simulink model "21-E"  (R2014a)
settings: Solver=FixedStepDiscrete  StartTime=0.0  StopTime=10.0  FixedStep=0.0005  RelTol=1e-3
undefined symbols (not defined in the file): add_k1_100, add_k2_100, ADDspeed, cal_acc_div, cal_acc_flo_add, cal_acc_min, cal_an_div, cal_an_min, cal_bre_div, cal_bre_en_add, cal_bre_flo_add, cal_bre_min, cal_conf_off, cal_conf_on, controller, ecucoder_acal, enres_on_add, enres_per_add
libraries: simulink x165, ec55xxlib x29
(part 2 of 6)

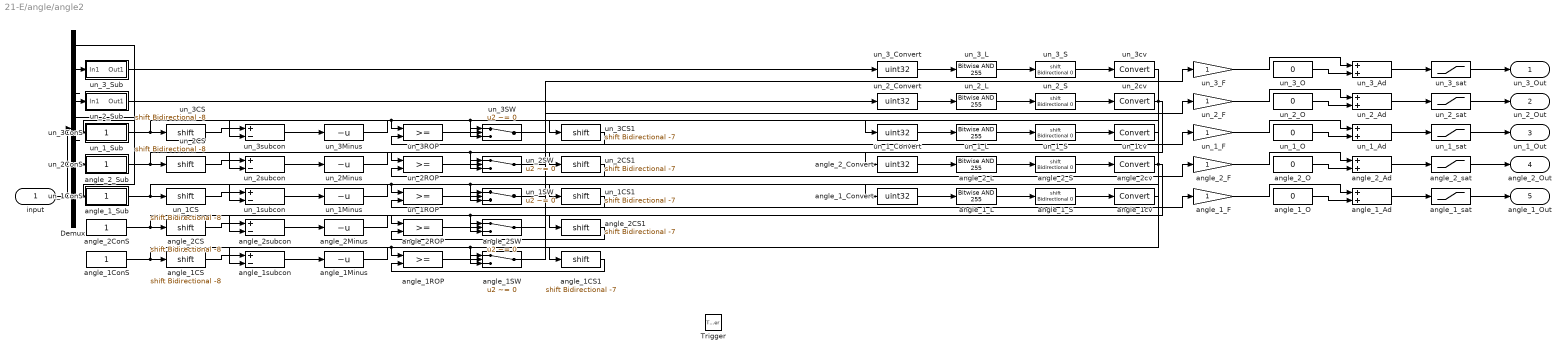
== system 21-E/angle/angle2 ==
  input : Inport
  Trigger : TriggerPort  TriggerType=function-call  PortDimensions=1
  Demux : Demux  Outputs=8
  angle_1CS : ArithShift  BitShiftNumber=-8
  angle_1CS1 : ArithShift  BitShiftNumber=-7
  angle_1ConS : Constant  OutDataTypeStr=single
  angle_1Minus : UnaryMinus
  angle_1ROP : RelationalOperator  OutDataTypeStr=boolean
  angle_1SW : Switch  Criteria=u2 ~= 0
  angle_1_Ad : Sum
  angle_1_Convert : DataTypeConversion  OutDataTypeStr=uint32
  angle_1_F : Gain
  angle_1_L : simulink/Logic and Bit Operations/Bitwise Operator  logicop=AND  UseBitMask=on  BitMask=255  BitMaskRealWorld=Stored Integer
  angle_1_O : Constant  Value=0  OutDataTypeStr=single
  angle_1_S : ArithShift
  angle_1_Sub : Subsystem
  angle_1_sat : Saturate  UpperLimit=255  LowerLimit=0
  angle_1cv : DataTypeConversion
  angle_1subcon : Sum  Inputs=+-
  angle_2CS : ArithShift  BitShiftNumber=-8
  angle_2CS1 : ArithShift  BitShiftNumber=-7
  angle_2ConS : Constant  OutDataTypeStr=single
  angle_2Minus : UnaryMinus
  angle_2ROP : RelationalOperator  OutDataTypeStr=boolean
  angle_2SW : Switch  Criteria=u2 ~= 0
  angle_2_Ad : Sum
  angle_2_Convert : DataTypeConversion  OutDataTypeStr=uint32
  angle_2_F : Gain
  angle_2_L : simulink/Logic and Bit Operations/Bitwise Operator  logicop=AND  UseBitMask=on  BitMask=255  BitMaskRealWorld=Stored Integer
  angle_2_O : Constant  Value=0  OutDataTypeStr=single
  angle_2_S : ArithShift
  angle_2_Sub : Subsystem
  angle_2_sat : Saturate  UpperLimit=255  LowerLimit=0
  angle_2cv : DataTypeConversion
  angle_2subcon : Sum  Inputs=+-
  un_1CS : ArithShift  BitShiftNumber=-8
  un_1CS1 : ArithShift  BitShiftNumber=-7
  un_1ConS : Constant  OutDataTypeStr=single
  un_1Minus : UnaryMinus
  un_1ROP : RelationalOperator  OutDataTypeStr=boolean
  un_1SW : Switch  Criteria=u2 ~= 0
  un_1_Ad : Sum
  un_1_Convert : DataTypeConversion  OutDataTypeStr=uint32
  un_1_F : Gain
  un_1_L : simulink/Logic and Bit Operations/Bitwise Operator  logicop=AND  UseBitMask=on  BitMask=255  BitMaskRealWorld=Stored Integer
  un_1_O : Constant  Value=0  OutDataTypeStr=single
  un_1_S : ArithShift
  un_1_Sub : Subsystem
  un_1_sat : Saturate  UpperLimit=255  LowerLimit=0
  un_1cv : DataTypeConversion
  un_1subcon : Sum  Inputs=+-
  un_2CS : ArithShift  BitShiftNumber=-8
  un_2CS1 : ArithShift  BitShiftNumber=-7
  un_2ConS : Constant  OutDataTypeStr=single
  un_2Minus : UnaryMinus
  un_2ROP : RelationalOperator  OutDataTypeStr=boolean
  un_2SW : Switch  Criteria=u2 ~= 0
  un_2_Ad : Sum
  un_2_Convert : DataTypeConversion  OutDataTypeStr=uint32
  un_2_F : Gain
  un_2_L : simulink/Logic and Bit Operations/Bitwise Operator  logicop=AND  UseBitMask=on  BitMask=255  BitMaskRealWorld=Stored Integer
  un_2_O : Constant  Value=0  OutDataTypeStr=single
  un_2_S : ArithShift
  un_2_Sub : Subsystem
  un_2_sat : Saturate  UpperLimit=255  LowerLimit=0
  un_2cv : DataTypeConversion
  un_2subcon : Sum  Inputs=+-
  un_3CS : ArithShift  BitShiftNumber=-8
  un_3CS1 : ArithShift  BitShiftNumber=-7
  un_3ConS : Constant  OutDataTypeStr=single
  un_3Minus : UnaryMinus
  un_3ROP : RelationalOperator  OutDataTypeStr=boolean
  un_3SW : Switch  Criteria=u2 ~= 0
  un_3_Ad : Sum
  un_3_Convert : DataTypeConversion  OutDataTypeStr=uint32
  un_3_F : Gain
  un_3_L : simulink/Logic and Bit Operations/Bitwise Operator  logicop=AND  UseBitMask=on  BitMask=255  BitMaskRealWorld=Stored Integer
  un_3_O : Constant  Value=0  OutDataTypeStr=single
  un_3_S : ArithShift
  un_3_Sub : Subsystem
  un_3_sat : Saturate  UpperLimit=255  LowerLimit=0
  un_3cv : DataTypeConversion
  un_3subcon : Sum  Inputs=+-
  un_3_Out : Outport
  un_2_Out : Outport  Port=2
  un_1_Out : Outport  Port=3
  angle_2_Out : Outport  Port=4
  angle_1_Out : Outport  Port=5
  wires:
  input/1 -> Demux/1
  angle_1ROP/1 -> angle_1SW/2
  angle_1SW/1 -> angle_1_F/1
  angle_1Minus/1 -> angle_1SW/1
  angle_1subcon/1 -> angle_1Minus/1
  angle_1CS/1 -> angle_1subcon/1
  angle_1CS1/1 -> angle_1ROP/2
  angle_1ConS/1 -> angle_1CS1/1, angle_1CS/1
  angle_1cv/1 -> angle_1subcon/2, angle_1ROP/1, angle_1SW/3
  angle_1_S/1 -> angle_1cv/1
  angle_1_L/1 -> angle_1_S/1
  angle_1_Convert/1 -> angle_1_L/1
  angle_1_Sub/1(Out1) -> angle_1_Convert/1
  Demux/4 -> angle_1_Sub/1(In1)
  angle_1_sat/1 -> angle_1_Out/1
  angle_1_Ad/1 -> angle_1_sat/1
  angle_1_O/1 -> angle_1_Ad/2
  angle_1_F/1 -> angle_1_Ad/1
  angle_2ROP/1 -> angle_2SW/2
  angle_2SW/1 -> angle_2_F/1
  angle_2Minus/1 -> angle_2SW/1
  angle_2subcon/1 -> angle_2Minus/1
  angle_2CS/1 -> angle_2subcon/1
  angle_2CS1/1 -> angle_2ROP/2
  angle_2ConS/1 -> angle_2CS1/1, angle_2CS/1
  angle_2cv/1 -> angle_2SW/3, angle_2subcon/2, angle_2ROP/1
  angle_2_S/1 -> angle_2cv/1
  angle_2_L/1 -> angle_2_S/1
  angle_2_Convert/1 -> angle_2_L/1
  angle_2_Sub/1(Out1) -> angle_2_Convert/1
  Demux/5 -> angle_2_Sub/1(In1)
  angle_2_sat/1 -> angle_2_Out/1
  angle_2_Ad/1 -> angle_2_sat/1
  angle_2_O/1 -> angle_2_Ad/2
  angle_2_F/1 -> angle_2_Ad/1
  un_1ROP/1 -> un_1SW/2
  un_1SW/1 -> un_1_F/1
  un_1Minus/1 -> un_1SW/1
  un_1subcon/1 -> un_1Minus/1
  un_1CS/1 -> un_1subcon/1
  un_1CS1/1 -> un_1ROP/2
  un_1ConS/1 -> un_1CS1/1, un_1CS/1
  un_1cv/1 -> un_1subcon/2, un_1ROP/1, un_1SW/3
  un_1_S/1 -> un_1cv/1
  un_1_L/1 -> un_1_S/1
  un_1_Convert/1 -> un_1_L/1
  un_1_Sub/1(Out1) -> un_1_Convert/1
  Demux/1 -> un_1_Sub/1(In1)
  un_1_sat/1 -> un_1_Out/1
  un_1_Ad/1 -> un_1_sat/1
  un_1_O/1 -> un_1_Ad/2
  un_1_F/1 -> un_1_Ad/1
  un_2ROP/1 -> un_2SW/2
  un_2SW/1 -> un_2_F/1
  un_2Minus/1 -> un_2SW/1
  un_2subcon/1 -> un_2Minus/1
  un_2CS/1 -> un_2subcon/1
  un_2CS1/1 -> un_2ROP/2
  un_2ConS/1 -> un_2CS1/1, un_2CS/1
  un_2cv/1 -> un_2SW/3, un_2subcon/2, un_2ROP/1
  un_2_S/1 -> un_2cv/1
  un_2_L/1 -> un_2_S/1
  un_2_Convert/1 -> un_2_L/1
  un_2_Sub/1(Out1) -> un_2_Convert/1
  Demux/2 -> un_2_Sub/1(In1)
  un_2_sat/1 -> un_2_Out/1
  un_2_Ad/1 -> un_2_sat/1
  un_2_O/1 -> un_2_Ad/2
  un_2_F/1 -> un_2_Ad/1
  un_3ROP/1 -> un_3SW/2
  un_3SW/1 -> un_3_F/1
  un_3Minus/1 -> un_3SW/1
  un_3subcon/1 -> un_3Minus/1
  un_3CS/1 -> un_3subcon/1
  un_3CS1/1 -> un_3ROP/2
  un_3ConS/1 -> un_3CS1/1, un_3CS/1
  un_3cv/1 -> un_3subcon/2, un_3ROP/1, un_3SW/3
  un_3_S/1 -> un_3cv/1
  un_3_L/1 -> un_3_S/1
  un_3_Convert/1 -> un_3_L/1
  un_3_Sub/1(Out1) -> un_3_Convert/1
  Demux/3 -> un_3_Sub/1(In1)
  un_3_sat/1 -> un_3_Out/1
  un_3_Ad/1 -> un_3_sat/1
  un_3_O/1 -> un_3_Ad/2
  un_3_F/1 -> un_3_Ad/1

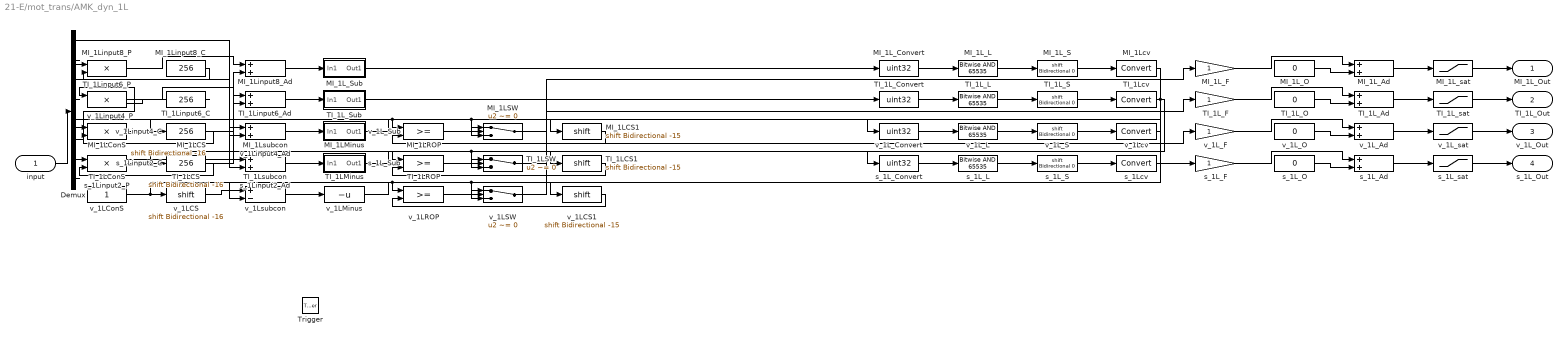
== system 21-E/mot_trans/AMK_dyn_1L ==
  input : Inport
  Trigger : TriggerPort  TriggerType=function-call  PortDimensions=1
  Demux : Demux  Outputs=8
  MI_1LCS : ArithShift  BitShiftNumber=-16
  MI_1LCS1 : ArithShift  BitShiftNumber=-15
  MI_1LConS : Constant  OutDataTypeStr=single
  MI_1LMinus : UnaryMinus
  MI_1LROP : RelationalOperator  OutDataTypeStr=boolean
  MI_1LSW : Switch  Criteria=u2 ~= 0
  MI_1L_Ad : Sum
  MI_1L_Convert : DataTypeConversion  OutDataTypeStr=uint32
  MI_1L_F : Gain
  MI_1L_L : simulink/Logic and Bit Operations/Bitwise Operator  logicop=AND  UseBitMask=on  BitMask=65535  BitMaskRealWorld=Stored Integer
  MI_1L_O : Constant  Value=0  OutDataTypeStr=single
  MI_1L_S : ArithShift
  MI_1L_Sub : Subsystem
  MI_1L_sat : Saturate  UpperLimit=32767  LowerLimit=-32768
  MI_1Lcv : DataTypeConversion
  MI_1Linput8_Ad : Sum
  MI_1Linput8_C : Constant  Value=256
  MI_1Linput8_P : Product
  MI_1Lsubcon : Sum  Inputs=+-
  TI_1LCS : ArithShift  BitShiftNumber=-16
  TI_1LCS1 : ArithShift  BitShiftNumber=-15
  TI_1LConS : Constant  OutDataTypeStr=single
  TI_1LMinus : UnaryMinus
  TI_1LROP : RelationalOperator  OutDataTypeStr=boolean
  TI_1LSW : Switch  Criteria=u2 ~= 0
  TI_1L_Ad : Sum
  TI_1L_Convert : DataTypeConversion  OutDataTypeStr=uint32
  TI_1L_F : Gain
  TI_1L_L : simulink/Logic and Bit Operations/Bitwise Operator  logicop=AND  UseBitMask=on  BitMask=65535  BitMaskRealWorld=Stored Integer
  TI_1L_O : Constant  Value=0  OutDataTypeStr=single
  TI_1L_S : ArithShift
  TI_1L_Sub : Subsystem
  TI_1L_sat : Saturate  UpperLimit=32767  LowerLimit=-32768
  TI_1Lcv : DataTypeConversion
  TI_1Linput6_Ad : Sum
  TI_1Linput6_C : Constant  Value=256
  TI_1Linput6_P : Product
  TI_1Lsubcon : Sum  Inputs=+-
  s_1L_Ad : Sum
  s_1L_Convert : DataTypeConversion  OutDataTypeStr=uint32
  s_1L_F : Gain
  s_1L_L : simulink/Logic and Bit Operations/Bitwise Operator  logicop=AND  UseBitMask=on  BitMask=65535  BitMaskRealWorld=Stored Integer
  s_1L_O : Constant  Value=0  OutDataTypeStr=single
  s_1L_S : ArithShift
  s_1L_Sub : Subsystem
  s_1L_sat : Saturate  UpperLimit=65535  LowerLimit=0
  s_1Lcv : DataTypeConversion
  s_1Linput2_Ad : Sum
  s_1Linput2_C : Constant  Value=256
  s_1Linput2_P : Product
  v_1LCS : ArithShift  BitShiftNumber=-16
  v_1LCS1 : ArithShift  BitShiftNumber=-15
  v_1LConS : Constant  OutDataTypeStr=single
  v_1LMinus : UnaryMinus
  v_1LROP : RelationalOperator  OutDataTypeStr=boolean
  v_1LSW : Switch  Criteria=u2 ~= 0
  v_1L_Ad : Sum
  v_1L_Convert : DataTypeConversion  OutDataTypeStr=uint32
  v_1L_F : Gain
  v_1L_L : simulink/Logic and Bit Operations/Bitwise Operator  logicop=AND  UseBitMask=on  BitMask=65535  BitMaskRealWorld=Stored Integer
  v_1L_O : Constant  Value=0  OutDataTypeStr=single
  v_1L_S : ArithShift
  v_1L_Sub : Subsystem
  v_1L_sat : Saturate  UpperLimit=32767  LowerLimit=-32768
  v_1Lcv : DataTypeConversion
  v_1Linput4_Ad : Sum
  v_1Linput4_C : Constant  Value=256
  v_1Linput4_P : Product
  v_1Lsubcon : Sum  Inputs=+-
  MI_1L_Out : Outport
  TI_1L_Out : Outport  Port=2
  v_1L_Out : Outport  Port=3
  s_1L_Out : Outport  Port=4
  wires:
  input/1 -> Demux/1
  s_1Lcv/1 -> s_1L_F/1
  s_1L_S/1 -> s_1Lcv/1
  s_1L_L/1 -> s_1L_S/1
  s_1L_Convert/1 -> s_1L_L/1
  s_1L_Sub/1(Out1) -> s_1L_Convert/1
  s_1Linput2_Ad/1 -> s_1L_Sub/1(In1)
  Demux/1 -> s_1Linput2_Ad/2
  s_1Linput2_P/1 -> s_1Linput2_Ad/1
  s_1Linput2_C/1 -> s_1Linput2_P/2
  Demux/2 -> s_1Linput2_P/1
  s_1L_sat/1 -> s_1L_Out/1
  s_1L_Ad/1 -> s_1L_sat/1
  s_1L_O/1 -> s_1L_Ad/2
  s_1L_F/1 -> s_1L_Ad/1
  v_1LROP/1 -> v_1LSW/2
  v_1LSW/1 -> v_1L_F/1
  v_1LMinus/1 -> v_1LSW/1
  v_1Lsubcon/1 -> v_1LMinus/1
  v_1LCS/1 -> v_1Lsubcon/1
  v_1LCS1/1 -> v_1LROP/2
  v_1LConS/1 -> v_1LCS1/1, v_1LCS/1
  v_1Lcv/1 -> v_1Lsubcon/2, v_1LROP/1, v_1LSW/3
  v_1L_S/1 -> v_1Lcv/1
  v_1L_L/1 -> v_1L_S/1
  v_1L_Convert/1 -> v_1L_L/1
  v_1L_Sub/1(Out1) -> v_1L_Convert/1
  v_1Linput4_Ad/1 -> v_1L_Sub/1(In1)
  Demux/3 -> v_1Linput4_Ad/2
  v_1Linput4_P/1 -> v_1Linput4_Ad/1
  v_1Linput4_C/1 -> v_1Linput4_P/2
  Demux/4 -> v_1Linput4_P/1
  v_1L_sat/1 -> v_1L_Out/1
  v_1L_Ad/1 -> v_1L_sat/1
  v_1L_O/1 -> v_1L_Ad/2
  v_1L_F/1 -> v_1L_Ad/1
  TI_1LROP/1 -> TI_1LSW/2
  TI_1LSW/1 -> TI_1L_F/1
  TI_1LMinus/1 -> TI_1LSW/1
  TI_1Lsubcon/1 -> TI_1LMinus/1
  TI_1LCS/1 -> TI_1Lsubcon/1
  TI_1LCS1/1 -> TI_1LROP/2
  TI_1LConS/1 -> TI_1LCS1/1, TI_1LCS/1
  TI_1Lcv/1 -> TI_1LSW/3, TI_1Lsubcon/2, TI_1LROP/1
  TI_1L_S/1 -> TI_1Lcv/1
  TI_1L_L/1 -> TI_1L_S/1
  TI_1L_Convert/1 -> TI_1L_L/1
  TI_1L_Sub/1(Out1) -> TI_1L_Convert/1
  TI_1Linput6_Ad/1 -> TI_1L_Sub/1(In1)
  Demux/5 -> TI_1Linput6_Ad/2
  TI_1Linput6_P/1 -> TI_1Linput6_Ad/1
  TI_1Linput6_C/1 -> TI_1Linput6_P/2
  Demux/6 -> TI_1Linput6_P/1
  TI_1L_sat/1 -> TI_1L_Out/1
  TI_1L_Ad/1 -> TI_1L_sat/1
  TI_1L_O/1 -> TI_1L_Ad/2
  TI_1L_F/1 -> TI_1L_Ad/1
  MI_1LROP/1 -> MI_1LSW/2
  MI_1LSW/1 -> MI_1L_F/1
  MI_1LMinus/1 -> MI_1LSW/1
  MI_1Lsubcon/1 -> MI_1LMinus/1
  MI_1LCS/1 -> MI_1Lsubcon/1
  MI_1LCS1/1 -> MI_1LROP/2
  MI_1LConS/1 -> MI_1LCS1/1, MI_1LCS/1
  MI_1Lcv/1 -> MI_1Lsubcon/2, MI_1LROP/1, MI_1LSW/3
  MI_1L_S/1 -> MI_1Lcv/1
  MI_1L_L/1 -> MI_1L_S/1
  MI_1L_Convert/1 -> MI_1L_L/1
  MI_1L_Sub/1(Out1) -> MI_1L_Convert/1
  MI_1Linput8_Ad/1 -> MI_1L_Sub/1(In1)
  Demux/7 -> MI_1Linput8_Ad/2
  MI_1Linput8_P/1 -> MI_1Linput8_Ad/1
  MI_1Linput8_C/1 -> MI_1Linput8_P/2
  Demux/8 -> MI_1Linput8_P/1
  MI_1L_sat/1 -> MI_1L_Out/1
  MI_1L_Ad/1 -> MI_1L_sat/1
  MI_1L_O/1 -> MI_1L_Ad/2
  MI_1L_F/1 -> MI_1L_Ad/1

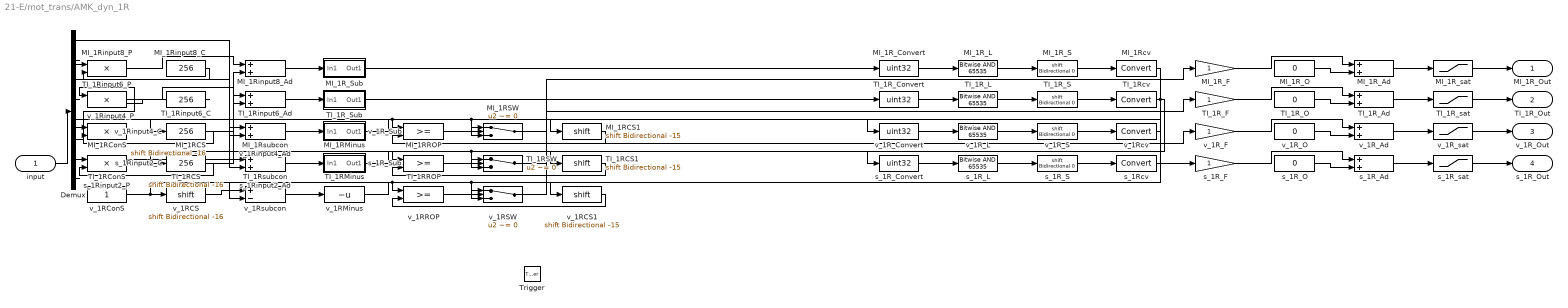
== system 21-E/mot_trans/AMK_dyn_1R ==
  input : Inport
  Trigger : TriggerPort  TriggerType=function-call  PortDimensions=1
  Demux : Demux  Outputs=8
  MI_1RCS : ArithShift  BitShiftNumber=-16
  MI_1RCS1 : ArithShift  BitShiftNumber=-15
  MI_1RConS : Constant  OutDataTypeStr=single
  MI_1RMinus : UnaryMinus
  MI_1RROP : RelationalOperator  OutDataTypeStr=boolean
  MI_1RSW : Switch  Criteria=u2 ~= 0
  MI_1R_Ad : Sum
  MI_1R_Convert : DataTypeConversion  OutDataTypeStr=uint32
  MI_1R_F : Gain
  MI_1R_L : simulink/Logic and Bit Operations/Bitwise Operator  logicop=AND  UseBitMask=on  BitMask=65535  BitMaskRealWorld=Stored Integer
  MI_1R_O : Constant  Value=0  OutDataTypeStr=single
  MI_1R_S : ArithShift
  MI_1R_Sub : Subsystem
  MI_1R_sat : Saturate  UpperLimit=32767  LowerLimit=-32768
  MI_1Rcv : DataTypeConversion
  MI_1Rinput8_Ad : Sum
  MI_1Rinput8_C : Constant  Value=256
  MI_1Rinput8_P : Product
  MI_1Rsubcon : Sum  Inputs=+-
  TI_1RCS : ArithShift  BitShiftNumber=-16
  TI_1RCS1 : ArithShift  BitShiftNumber=-15
  TI_1RConS : Constant  OutDataTypeStr=single
  TI_1RMinus : UnaryMinus
  TI_1RROP : RelationalOperator  OutDataTypeStr=boolean
  TI_1RSW : Switch  Criteria=u2 ~= 0
  TI_1R_Ad : Sum
  TI_1R_Convert : DataTypeConversion  OutDataTypeStr=uint32
  TI_1R_F : Gain
  TI_1R_L : simulink/Logic and Bit Operations/Bitwise Operator  logicop=AND  UseBitMask=on  BitMask=65535  BitMaskRealWorld=Stored Integer
  TI_1R_O : Constant  Value=0  OutDataTypeStr=single
  TI_1R_S : ArithShift
  TI_1R_Sub : Subsystem
  TI_1R_sat : Saturate  UpperLimit=32767  LowerLimit=-32768
  TI_1Rcv : DataTypeConversion
  TI_1Rinput6_Ad : Sum
  TI_1Rinput6_C : Constant  Value=256
  TI_1Rinput6_P : Product
  TI_1Rsubcon : Sum  Inputs=+-
  s_1R_Ad : Sum
  s_1R_Convert : DataTypeConversion  OutDataTypeStr=uint32
  s_1R_F : Gain
  s_1R_L : simulink/Logic and Bit Operations/Bitwise Operator  logicop=AND  UseBitMask=on  BitMask=65535  BitMaskRealWorld=Stored Integer
  s_1R_O : Constant  Value=0  OutDataTypeStr=single
  s_1R_S : ArithShift
  s_1R_Sub : Subsystem
  s_1R_sat : Saturate  UpperLimit=65535  LowerLimit=0
  s_1Rcv : DataTypeConversion
  s_1Rinput2_Ad : Sum
  s_1Rinput2_C : Constant  Value=256
  s_1Rinput2_P : Product
  v_1RCS : ArithShift  BitShiftNumber=-16
  v_1RCS1 : ArithShift  BitShiftNumber=-15
  v_1RConS : Constant  OutDataTypeStr=single
  v_1RMinus : UnaryMinus
  v_1RROP : RelationalOperator  OutDataTypeStr=boolean
  v_1RSW : Switch  Criteria=u2 ~= 0
  v_1R_Ad : Sum
  v_1R_Convert : DataTypeConversion  OutDataTypeStr=uint32
  v_1R_F : Gain
  v_1R_L : simulink/Logic and Bit Operations/Bitwise Operator  logicop=AND  UseBitMask=on  BitMask=65535  BitMaskRealWorld=Stored Integer
  v_1R_O : Constant  Value=0  OutDataTypeStr=single
  v_1R_S : ArithShift
  v_1R_Sub : Subsystem
  v_1R_sat : Saturate  UpperLimit=32767  LowerLimit=-32768
  v_1Rcv : DataTypeConversion
  v_1Rinput4_Ad : Sum
  v_1Rinput4_C : Constant  Value=256
  v_1Rinput4_P : Product
  v_1Rsubcon : Sum  Inputs=+-
  MI_1R_Out : Outport
  TI_1R_Out : Outport  Port=2
  v_1R_Out : Outport  Port=3
  s_1R_Out : Outport  Port=4
  wires:
  input/1 -> Demux/1
  s_1Rcv/1 -> s_1R_F/1
  s_1R_S/1 -> s_1Rcv/1
  s_1R_L/1 -> s_1R_S/1
  s_1R_Convert/1 -> s_1R_L/1
  s_1R_Sub/1(Out1) -> s_1R_Convert/1
  s_1Rinput2_Ad/1 -> s_1R_Sub/1(In1)
  Demux/1 -> s_1Rinput2_Ad/2
  s_1Rinput2_P/1 -> s_1Rinput2_Ad/1
  s_1Rinput2_C/1 -> s_1Rinput2_P/2
  Demux/2 -> s_1Rinput2_P/1
  s_1R_sat/1 -> s_1R_Out/1
  s_1R_Ad/1 -> s_1R_sat/1
  s_1R_O/1 -> s_1R_Ad/2
  s_1R_F/1 -> s_1R_Ad/1
  v_1RROP/1 -> v_1RSW/2
  v_1RSW/1 -> v_1R_F/1
  v_1RMinus/1 -> v_1RSW/1
  v_1Rsubcon/1 -> v_1RMinus/1
  v_1RCS/1 -> v_1Rsubcon/1
  v_1RCS1/1 -> v_1RROP/2
  v_1RConS/1 -> v_1RCS1/1, v_1RCS/1
  v_1Rcv/1 -> v_1Rsubcon/2, v_1RROP/1, v_1RSW/3
  v_1R_S/1 -> v_1Rcv/1
  v_1R_L/1 -> v_1R_S/1
  v_1R_Convert/1 -> v_1R_L/1
  v_1R_Sub/1(Out1) -> v_1R_Convert/1
  v_1Rinput4_Ad/1 -> v_1R_Sub/1(In1)
  Demux/3 -> v_1Rinput4_Ad/2
  v_1Rinput4_P/1 -> v_1Rinput4_Ad/1
  v_1Rinput4_C/1 -> v_1Rinput4_P/2
  Demux/4 -> v_1Rinput4_P/1
  v_1R_sat/1 -> v_1R_Out/1
  v_1R_Ad/1 -> v_1R_sat/1
  v_1R_O/1 -> v_1R_Ad/2
  v_1R_F/1 -> v_1R_Ad/1
  TI_1RROP/1 -> TI_1RSW/2
  TI_1RSW/1 -> TI_1R_F/1
  TI_1RMinus/1 -> TI_1RSW/1
  TI_1Rsubcon/1 -> TI_1RMinus/1
  TI_1RCS/1 -> TI_1Rsubcon/1
  TI_1RCS1/1 -> TI_1RROP/2
  TI_1RConS/1 -> TI_1RCS1/1, TI_1RCS/1
  TI_1Rcv/1 -> TI_1RSW/3, TI_1Rsubcon/2, TI_1RROP/1
  TI_1R_S/1 -> TI_1Rcv/1
  TI_1R_L/1 -> TI_1R_S/1
  TI_1R_Convert/1 -> TI_1R_L/1
  TI_1R_Sub/1(Out1) -> TI_1R_Convert/1
  TI_1Rinput6_Ad/1 -> TI_1R_Sub/1(In1)
  Demux/5 -> TI_1Rinput6_Ad/2
  TI_1Rinput6_P/1 -> TI_1Rinput6_Ad/1
  TI_1Rinput6_C/1 -> TI_1Rinput6_P/2
  Demux/6 -> TI_1Rinput6_P/1
  TI_1R_sat/1 -> TI_1R_Out/1
  TI_1R_Ad/1 -> TI_1R_sat/1
  TI_1R_O/1 -> TI_1R_Ad/2
  TI_1R_F/1 -> TI_1R_Ad/1
  MI_1RROP/1 -> MI_1RSW/2
  MI_1RSW/1 -> MI_1R_F/1
  MI_1RMinus/1 -> MI_1RSW/1
  MI_1Rsubcon/1 -> MI_1RMinus/1
  MI_1RCS/1 -> MI_1Rsubcon/1
  MI_1RCS1/1 -> MI_1RROP/2
  MI_1RConS/1 -> MI_1RCS1/1, MI_1RCS/1
  MI_1Rcv/1 -> MI_1Rsubcon/2, MI_1RROP/1, MI_1RSW/3
  MI_1R_S/1 -> MI_1Rcv/1
  MI_1R_L/1 -> MI_1R_S/1
  MI_1R_Convert/1 -> MI_1R_L/1
  MI_1R_Sub/1(Out1) -> MI_1R_Convert/1
  MI_1Rinput8_Ad/1 -> MI_1R_Sub/1(In1)
  Demux/7 -> MI_1Rinput8_Ad/2
  MI_1Rinput8_P/1 -> MI_1Rinput8_Ad/1
  MI_1Rinput8_C/1 -> MI_1Rinput8_P/2
  Demux/8 -> MI_1Rinput8_P/1
  MI_1R_sat/1 -> MI_1R_Out/1
  MI_1R_Ad/1 -> MI_1R_sat/1
  MI_1R_O/1 -> MI_1R_Ad/2
  MI_1R_F/1 -> MI_1R_Ad/1

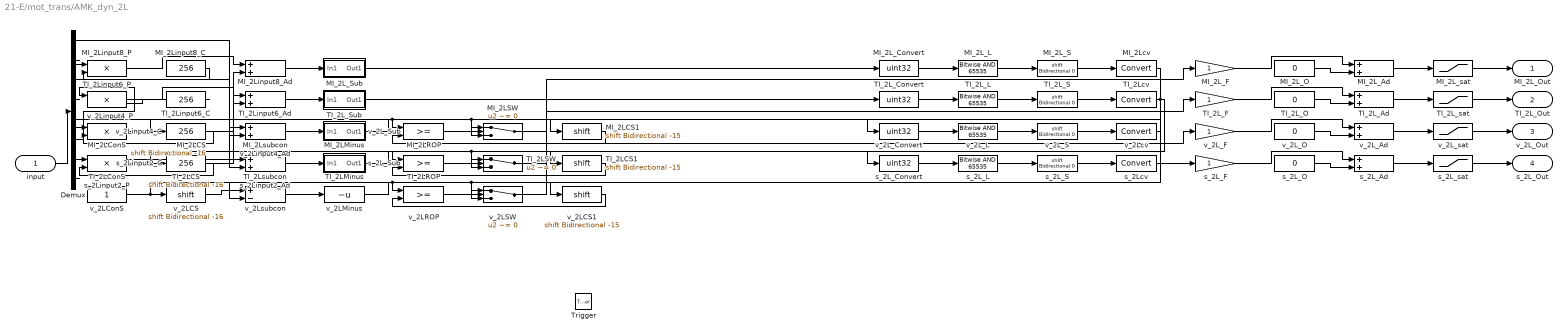
== system 21-E/mot_trans/AMK_dyn_2L ==
  input : Inport
  Trigger : TriggerPort  TriggerType=function-call  PortDimensions=1
  Demux : Demux  Outputs=8
  MI_2LCS : ArithShift  BitShiftNumber=-16
  MI_2LCS1 : ArithShift  BitShiftNumber=-15
  MI_2LConS : Constant  OutDataTypeStr=single
  MI_2LMinus : UnaryMinus
  MI_2LROP : RelationalOperator  OutDataTypeStr=boolean
  MI_2LSW : Switch  Criteria=u2 ~= 0
  MI_2L_Ad : Sum
  MI_2L_Convert : DataTypeConversion  OutDataTypeStr=uint32
  MI_2L_F : Gain
  MI_2L_L : simulink/Logic and Bit Operations/Bitwise Operator  logicop=AND  UseBitMask=on  BitMask=65535  BitMaskRealWorld=Stored Integer
  MI_2L_O : Constant  Value=0  OutDataTypeStr=single
  MI_2L_S : ArithShift
  MI_2L_Sub : Subsystem
  MI_2L_sat : Saturate  UpperLimit=32767  LowerLimit=-32768
  MI_2Lcv : DataTypeConversion
  MI_2Linput8_Ad : Sum
  MI_2Linput8_C : Constant  Value=256
  MI_2Linput8_P : Product
  MI_2Lsubcon : Sum  Inputs=+-
  TI_2LCS : ArithShift  BitShiftNumber=-16
  TI_2LCS1 : ArithShift  BitShiftNumber=-15
  TI_2LConS : Constant  OutDataTypeStr=single
  TI_2LMinus : UnaryMinus
  TI_2LROP : RelationalOperator  OutDataTypeStr=boolean
  TI_2LSW : Switch  Criteria=u2 ~= 0
  TI_2L_Ad : Sum
  TI_2L_Convert : DataTypeConversion  OutDataTypeStr=uint32
  TI_2L_F : Gain
  TI_2L_L : simulink/Logic and Bit Operations/Bitwise Operator  logicop=AND  UseBitMask=on  BitMask=65535  BitMaskRealWorld=Stored Integer
  TI_2L_O : Constant  Value=0  OutDataTypeStr=single
  TI_2L_S : ArithShift
  TI_2L_Sub : Subsystem
  TI_2L_sat : Saturate  UpperLimit=32767  LowerLimit=-32768
  TI_2Lcv : DataTypeConversion
  TI_2Linput6_Ad : Sum
  TI_2Linput6_C : Constant  Value=256
  TI_2Linput6_P : Product
  TI_2Lsubcon : Sum  Inputs=+-
  s_2L_Ad : Sum
  s_2L_Convert : DataTypeConversion  OutDataTypeStr=uint32
  s_2L_F : Gain
  s_2L_L : simulink/Logic and Bit Operations/Bitwise Operator  logicop=AND  UseBitMask=on  BitMask=65535  BitMaskRealWorld=Stored Integer
  s_2L_O : Constant  Value=0  OutDataTypeStr=single
  s_2L_S : ArithShift
  s_2L_Sub : Subsystem
  s_2L_sat : Saturate  UpperLimit=65535  LowerLimit=0
  s_2Lcv : DataTypeConversion
  s_2Linput2_Ad : Sum
  s_2Linput2_C : Constant  Value=256
  s_2Linput2_P : Product
  v_2LCS : ArithShift  BitShiftNumber=-16
  v_2LCS1 : ArithShift  BitShiftNumber=-15
  v_2LConS : Constant  OutDataTypeStr=single
  v_2LMinus : UnaryMinus
  v_2LROP : RelationalOperator  OutDataTypeStr=boolean
  v_2LSW : Switch  Criteria=u2 ~= 0
  v_2L_Ad : Sum
  v_2L_Convert : DataTypeConversion  OutDataTypeStr=uint32
  v_2L_F : Gain
  v_2L_L : simulink/Logic and Bit Operations/Bitwise Operator  logicop=AND  UseBitMask=on  BitMask=65535  BitMaskRealWorld=Stored Integer
  v_2L_O : Constant  Value=0  OutDataTypeStr=single
  v_2L_S : ArithShift
  v_2L_Sub : Subsystem
  v_2L_sat : Saturate  UpperLimit=32767  LowerLimit=-32768
  v_2Lcv : DataTypeConversion
  v_2Linput4_Ad : Sum
  v_2Linput4_C : Constant  Value=256
  v_2Linput4_P : Product
  v_2Lsubcon : Sum  Inputs=+-
  MI_2L_Out : Outport
  TI_2L_Out : Outport  Port=2
  v_2L_Out : Outport  Port=3
  s_2L_Out : Outport  Port=4
  wires:
  input/1 -> Demux/1
  s_2Lcv/1 -> s_2L_F/1
  s_2L_S/1 -> s_2Lcv/1
  s_2L_L/1 -> s_2L_S/1
  s_2L_Convert/1 -> s_2L_L/1
  s_2L_Sub/1(Out1) -> s_2L_Convert/1
  s_2Linput2_Ad/1 -> s_2L_Sub/1(In1)
  Demux/1 -> s_2Linput2_Ad/2
  s_2Linput2_P/1 -> s_2Linput2_Ad/1
  s_2Linput2_C/1 -> s_2Linput2_P/2
  Demux/2 -> s_2Linput2_P/1
  s_2L_sat/1 -> s_2L_Out/1
  s_2L_Ad/1 -> s_2L_sat/1
  s_2L_O/1 -> s_2L_Ad/2
  s_2L_F/1 -> s_2L_Ad/1
  v_2LROP/1 -> v_2LSW/2
  v_2LSW/1 -> v_2L_F/1
  v_2LMinus/1 -> v_2LSW/1
  v_2Lsubcon/1 -> v_2LMinus/1
  v_2LCS/1 -> v_2Lsubcon/1
  v_2LCS1/1 -> v_2LROP/2
  v_2LConS/1 -> v_2LCS1/1, v_2LCS/1
  v_2Lcv/1 -> v_2Lsubcon/2, v_2LROP/1, v_2LSW/3
  v_2L_S/1 -> v_2Lcv/1
  v_2L_L/1 -> v_2L_S/1
  v_2L_Convert/1 -> v_2L_L/1
  v_2L_Sub/1(Out1) -> v_2L_Convert/1
  v_2Linput4_Ad/1 -> v_2L_Sub/1(In1)
  Demux/3 -> v_2Linput4_Ad/2
  v_2Linput4_P/1 -> v_2Linput4_Ad/1
  v_2Linput4_C/1 -> v_2Linput4_P/2
  Demux/4 -> v_2Linput4_P/1
  v_2L_sat/1 -> v_2L_Out/1
  v_2L_Ad/1 -> v_2L_sat/1
  v_2L_O/1 -> v_2L_Ad/2
  v_2L_F/1 -> v_2L_Ad/1
  TI_2LROP/1 -> TI_2LSW/2
  TI_2LSW/1 -> TI_2L_F/1
  TI_2LMinus/1 -> TI_2LSW/1
  TI_2Lsubcon/1 -> TI_2LMinus/1
  TI_2LCS/1 -> TI_2Lsubcon/1
  TI_2LCS1/1 -> TI_2LROP/2
  TI_2LConS/1 -> TI_2LCS1/1, TI_2LCS/1
  TI_2Lcv/1 -> TI_2LSW/3, TI_2Lsubcon/2, TI_2LROP/1
  TI_2L_S/1 -> TI_2Lcv/1
  TI_2L_L/1 -> TI_2L_S/1
  TI_2L_Convert/1 -> TI_2L_L/1
  TI_2L_Sub/1(Out1) -> TI_2L_Convert/1
  TI_2Linput6_Ad/1 -> TI_2L_Sub/1(In1)
  Demux/5 -> TI_2Linput6_Ad/2
  TI_2Linput6_P/1 -> TI_2Linput6_Ad/1
  TI_2Linput6_C/1 -> TI_2Linput6_P/2
  Demux/6 -> TI_2Linput6_P/1
  TI_2L_sat/1 -> TI_2L_Out/1
  TI_2L_Ad/1 -> TI_2L_sat/1
  TI_2L_O/1 -> TI_2L_Ad/2
  TI_2L_F/1 -> TI_2L_Ad/1
  MI_2LROP/1 -> MI_2LSW/2
  MI_2LSW/1 -> MI_2L_F/1
  MI_2LMinus/1 -> MI_2LSW/1
  MI_2Lsubcon/1 -> MI_2LMinus/1
  MI_2LCS/1 -> MI_2Lsubcon/1
  MI_2LCS1/1 -> MI_2LROP/2
  MI_2LConS/1 -> MI_2LCS1/1, MI_2LCS/1
  MI_2Lcv/1 -> MI_2Lsubcon/2, MI_2LROP/1, MI_2LSW/3
  MI_2L_S/1 -> MI_2Lcv/1
  MI_2L_L/1 -> MI_2L_S/1
  MI_2L_Convert/1 -> MI_2L_L/1
  MI_2L_Sub/1(Out1) -> MI_2L_Convert/1
  MI_2Linput8_Ad/1 -> MI_2L_Sub/1(In1)
  Demux/7 -> MI_2Linput8_Ad/2
  MI_2Linput8_P/1 -> MI_2Linput8_Ad/1
  MI_2Linput8_C/1 -> MI_2Linput8_P/2
  Demux/8 -> MI_2Linput8_P/1
  MI_2L_sat/1 -> MI_2L_Out/1
  MI_2L_Ad/1 -> MI_2L_sat/1
  MI_2L_O/1 -> MI_2L_Ad/2
  MI_2L_F/1 -> MI_2L_Ad/1

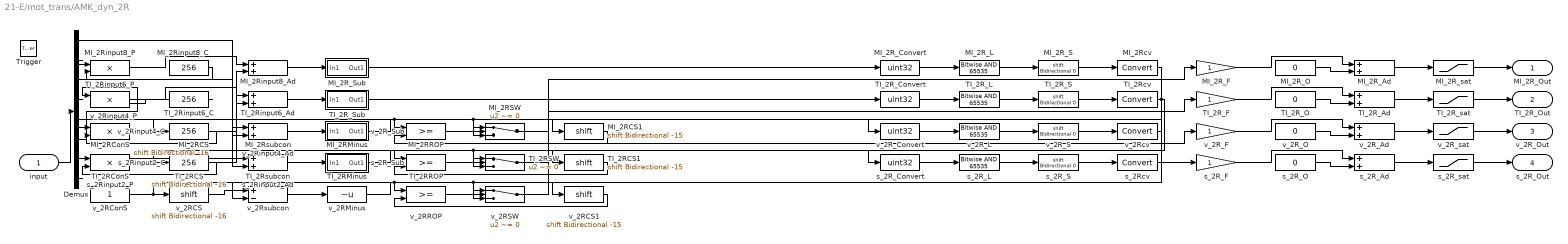
== system 21-E/mot_trans/AMK_dyn_2R ==
  input : Inport
  Trigger : TriggerPort  TriggerType=function-call  PortDimensions=1
  Demux : Demux  Outputs=8
  MI_2RCS : ArithShift  BitShiftNumber=-16
  MI_2RCS1 : ArithShift  BitShiftNumber=-15
  MI_2RConS : Constant  OutDataTypeStr=single
  MI_2RMinus : UnaryMinus
  MI_2RROP : RelationalOperator  OutDataTypeStr=boolean
  MI_2RSW : Switch  Criteria=u2 ~= 0
  MI_2R_Ad : Sum
  MI_2R_Convert : DataTypeConversion  OutDataTypeStr=uint32
  MI_2R_F : Gain
  MI_2R_L : simulink/Logic and Bit Operations/Bitwise Operator  logicop=AND  UseBitMask=on  BitMask=65535  BitMaskRealWorld=Stored Integer
  MI_2R_O : Constant  Value=0  OutDataTypeStr=single
  MI_2R_S : ArithShift
  MI_2R_Sub : Subsystem
  MI_2R_sat : Saturate  UpperLimit=32767  LowerLimit=-32768
  MI_2Rcv : DataTypeConversion
  MI_2Rinput8_Ad : Sum
  MI_2Rinput8_C : Constant  Value=256
  MI_2Rinput8_P : Product
  MI_2Rsubcon : Sum  Inputs=+-
  TI_2RCS : ArithShift  BitShiftNumber=-16
  TI_2RCS1 : ArithShift  BitShiftNumber=-15
  TI_2RConS : Constant  OutDataTypeStr=single
  TI_2RMinus : UnaryMinus
  TI_2RROP : RelationalOperator  OutDataTypeStr=boolean
  TI_2RSW : Switch  Criteria=u2 ~= 0
  TI_2R_Ad : Sum
  TI_2R_Convert : DataTypeConversion  OutDataTypeStr=uint32
  TI_2R_F : Gain
  TI_2R_L : simulink/Logic and Bit Operations/Bitwise Operator  logicop=AND  UseBitMask=on  BitMask=65535  BitMaskRealWorld=Stored Integer
  TI_2R_O : Constant  Value=0  OutDataTypeStr=single
  TI_2R_S : ArithShift
  TI_2R_Sub : Subsystem
  TI_2R_sat : Saturate  UpperLimit=32767  LowerLimit=-32768
  TI_2Rcv : DataTypeConversion
  TI_2Rinput6_Ad : Sum
  TI_2Rinput6_C : Constant  Value=256
  TI_2Rinput6_P : Product
  TI_2Rsubcon : Sum  Inputs=+-
  s_2R_Ad : Sum
  s_2R_Convert : DataTypeConversion  OutDataTypeStr=uint32
  s_2R_F : Gain
  s_2R_L : simulink/Logic and Bit Operations/Bitwise Operator  logicop=AND  UseBitMask=on  BitMask=65535  BitMaskRealWorld=Stored Integer
  s_2R_O : Constant  Value=0  OutDataTypeStr=single
  s_2R_S : ArithShift
  s_2R_Sub : Subsystem
  s_2R_sat : Saturate  UpperLimit=65535  LowerLimit=0
  s_2Rcv : DataTypeConversion
  s_2Rinput2_Ad : Sum
  s_2Rinput2_C : Constant  Value=256
  s_2Rinput2_P : Product
  v_2RCS : ArithShift  BitShiftNumber=-16
  v_2RCS1 : ArithShift  BitShiftNumber=-15
  v_2RConS : Constant  OutDataTypeStr=single
  v_2RMinus : UnaryMinus
  v_2RROP : RelationalOperator  OutDataTypeStr=boolean
  v_2RSW : Switch  Criteria=u2 ~= 0
  v_2R_Ad : Sum
  v_2R_Convert : DataTypeConversion  OutDataTypeStr=uint32
  v_2R_F : Gain
  v_2R_L : simulink/Logic and Bit Operations/Bitwise Operator  logicop=AND  UseBitMask=on  BitMask=65535  BitMaskRealWorld=Stored Integer
  v_2R_O : Constant  Value=0  OutDataTypeStr=single
  v_2R_S : ArithShift
  v_2R_Sub : Subsystem
  v_2R_sat : Saturate  UpperLimit=32767  LowerLimit=-32768
  v_2Rcv : DataTypeConversion
  v_2Rinput4_Ad : Sum
  v_2Rinput4_C : Constant  Value=256
  v_2Rinput4_P : Product
  v_2Rsubcon : Sum  Inputs=+-
  MI_2R_Out : Outport
  TI_2R_Out : Outport  Port=2
  v_2R_Out : Outport  Port=3
  s_2R_Out : Outport  Port=4
  wires:
  input/1 -> Demux/1
  s_2Rcv/1 -> s_2R_F/1
  s_2R_S/1 -> s_2Rcv/1
  s_2R_L/1 -> s_2R_S/1
  s_2R_Convert/1 -> s_2R_L/1
  s_2R_Sub/1(Out1) -> s_2R_Convert/1
  s_2Rinput2_Ad/1 -> s_2R_Sub/1(In1)
  Demux/1 -> s_2Rinput2_Ad/2
  s_2Rinput2_P/1 -> s_2Rinput2_Ad/1
  s_2Rinput2_C/1 -> s_2Rinput2_P/2
  Demux/2 -> s_2Rinput2_P/1
  s_2R_sat/1 -> s_2R_Out/1
  s_2R_Ad/1 -> s_2R_sat/1
  s_2R_O/1 -> s_2R_Ad/2
  s_2R_F/1 -> s_2R_Ad/1
  v_2RROP/1 -> v_2RSW/2
  v_2RSW/1 -> v_2R_F/1
  v_2RMinus/1 -> v_2RSW/1
  v_2Rsubcon/1 -> v_2RMinus/1
  v_2RCS/1 -> v_2Rsubcon/1
  v_2RCS1/1 -> v_2RROP/2
  v_2RConS/1 -> v_2RCS1/1, v_2RCS/1
  v_2Rcv/1 -> v_2Rsubcon/2, v_2RROP/1, v_2RSW/3
  v_2R_S/1 -> v_2Rcv/1
  v_2R_L/1 -> v_2R_S/1
  v_2R_Convert/1 -> v_2R_L/1
  v_2R_Sub/1(Out1) -> v_2R_Convert/1
  v_2Rinput4_Ad/1 -> v_2R_Sub/1(In1)
  Demux/3 -> v_2Rinput4_Ad/2
  v_2Rinput4_P/1 -> v_2Rinput4_Ad/1
  v_2Rinput4_C/1 -> v_2Rinput4_P/2
  Demux/4 -> v_2Rinput4_P/1
  v_2R_sat/1 -> v_2R_Out/1
  v_2R_Ad/1 -> v_2R_sat/1
  v_2R_O/1 -> v_2R_Ad/2
  v_2R_F/1 -> v_2R_Ad/1
  TI_2RROP/1 -> TI_2RSW/2
  TI_2RSW/1 -> TI_2R_F/1
  TI_2RMinus/1 -> TI_2RSW/1
  TI_2Rsubcon/1 -> TI_2RMinus/1
  TI_2RCS/1 -> TI_2Rsubcon/1
  TI_2RCS1/1 -> TI_2RROP/2
  TI_2RConS/1 -> TI_2RCS1/1, TI_2RCS/1
  TI_2Rcv/1 -> TI_2RSW/3, TI_2Rsubcon/2, TI_2RROP/1
  TI_2R_S/1 -> TI_2Rcv/1
  TI_2R_L/1 -> TI_2R_S/1
  TI_2R_Convert/1 -> TI_2R_L/1
  TI_2R_Sub/1(Out1) -> TI_2R_Convert/1
  TI_2Rinput6_Ad/1 -> TI_2R_Sub/1(In1)
  Demux/5 -> TI_2Rinput6_Ad/2
  TI_2Rinput6_P/1 -> TI_2Rinput6_Ad/1
  TI_2Rinput6_C/1 -> TI_2Rinput6_P/2
  Demux/6 -> TI_2Rinput6_P/1
  TI_2R_sat/1 -> TI_2R_Out/1
  TI_2R_Ad/1 -> TI_2R_sat/1
  TI_2R_O/1 -> TI_2R_Ad/2
  TI_2R_F/1 -> TI_2R_Ad/1
  MI_2RROP/1 -> MI_2RSW/2
  MI_2RSW/1 -> MI_2R_F/1
  MI_2RMinus/1 -> MI_2RSW/1
  MI_2Rsubcon/1 -> MI_2RMinus/1
  MI_2RCS/1 -> MI_2Rsubcon/1
  MI_2RCS1/1 -> MI_2RROP/2
  MI_2RConS/1 -> MI_2RCS1/1, MI_2RCS/1
  MI_2Rcv/1 -> MI_2Rsubcon/2, MI_2RROP/1, MI_2RSW/3
  MI_2R_S/1 -> MI_2Rcv/1
  MI_2R_L/1 -> MI_2R_S/1
  MI_2R_Convert/1 -> MI_2R_L/1
  MI_2R_Sub/1(Out1) -> MI_2R_Convert/1
  MI_2Rinput8_Ad/1 -> MI_2R_Sub/1(In1)
  Demux/7 -> MI_2Rinput8_Ad/2
  MI_2Rinput8_P/1 -> MI_2Rinput8_Ad/1
  MI_2Rinput8_C/1 -> MI_2Rinput8_P/2
  Demux/8 -> MI_2Rinput8_P/1
  MI_2R_sat/1 -> MI_2R_Out/1
  MI_2R_Ad/1 -> MI_2R_sat/1
  MI_2R_O/1 -> MI_2R_Ad/2
  MI_2R_F/1 -> MI_2R_Ad/1

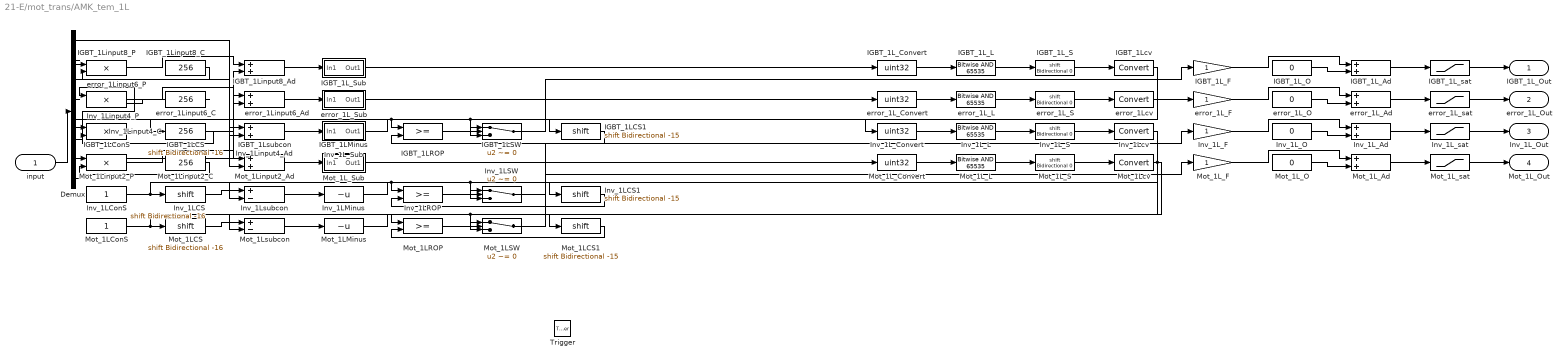
== system 21-E/mot_trans/AMK_tem_1L ==
  input : Inport
  Trigger : TriggerPort  TriggerType=function-call  PortDimensions=1
  Demux : Demux  Outputs=8
  IGBT_1LCS : ArithShift  BitShiftNumber=-16
  IGBT_1LCS1 : ArithShift  BitShiftNumber=-15
  IGBT_1LConS : Constant  OutDataTypeStr=single
  IGBT_1LMinus : UnaryMinus
  IGBT_1LROP : RelationalOperator  OutDataTypeStr=boolean
  IGBT_1LSW : Switch  Criteria=u2 ~= 0
  IGBT_1L_Ad : Sum
  IGBT_1L_Convert : DataTypeConversion  OutDataTypeStr=uint32
  IGBT_1L_F : Gain
  IGBT_1L_L : simulink/Logic and Bit Operations/Bitwise Operator  logicop=AND  UseBitMask=on  BitMask=65535  BitMaskRealWorld=Stored Integer
  IGBT_1L_O : Constant  Value=0  OutDataTypeStr=single
  IGBT_1L_S : ArithShift
  IGBT_1L_Sub : Subsystem
  IGBT_1L_sat : Saturate  UpperLimit=32767  LowerLimit=-32768
  IGBT_1Lcv : DataTypeConversion
  IGBT_1Linput8_Ad : Sum
  IGBT_1Linput8_C : Constant  Value=256
  IGBT_1Linput8_P : Product
  IGBT_1Lsubcon : Sum  Inputs=+-
  Inv_1LCS : ArithShift  BitShiftNumber=-16
  Inv_1LCS1 : ArithShift  BitShiftNumber=-15
  Inv_1LConS : Constant  OutDataTypeStr=single
  Inv_1LMinus : UnaryMinus
  Inv_1LROP : RelationalOperator  OutDataTypeStr=boolean
  Inv_1LSW : Switch  Criteria=u2 ~= 0
  Inv_1L_Ad : Sum
  Inv_1L_Convert : DataTypeConversion  OutDataTypeStr=uint32
  Inv_1L_F : Gain
  Inv_1L_L : simulink/Logic and Bit Operations/Bitwise Operator  logicop=AND  UseBitMask=on  BitMask=65535  BitMaskRealWorld=Stored Integer
  Inv_1L_O : Constant  Value=0  OutDataTypeStr=single
  Inv_1L_S : ArithShift
  Inv_1L_Sub : Subsystem
  Inv_1L_sat : Saturate  UpperLimit=32767  LowerLimit=-32768
  Inv_1Lcv : DataTypeConversion
  Inv_1Linput4_Ad : Sum
  Inv_1Linput4_C : Constant  Value=256
  Inv_1Linput4_P : Product
  Inv_1Lsubcon : Sum  Inputs=+-
  Mot_1LCS : ArithShift  BitShiftNumber=-16
  Mot_1LCS1 : ArithShift  BitShiftNumber=-15
  Mot_1LConS : Constant  OutDataTypeStr=single
  Mot_1LMinus : UnaryMinus
  Mot_1LROP : RelationalOperator  OutDataTypeStr=boolean
  Mot_1LSW : Switch  Criteria=u2 ~= 0
  Mot_1L_Ad : Sum
  Mot_1L_Convert : DataTypeConversion  OutDataTypeStr=uint32
  Mot_1L_F : Gain
  Mot_1L_L : simulink/Logic and Bit Operations/Bitwise Operator  logicop=AND  UseBitMask=on  BitMask=65535  BitMaskRealWorld=Stored Integer
  Mot_1L_O : Constant  Value=0  OutDataTypeStr=single
  Mot_1L_S : ArithShift
  Mot_1L_Sub : Subsystem
  Mot_1L_sat : Saturate  UpperLimit=32767  LowerLimit=-32768
  Mot_1Lcv : DataTypeConversion
  Mot_1Linput2_Ad : Sum
  Mot_1Linput2_C : Constant  Value=256
  Mot_1Linput2_P : Product
  Mot_1Lsubcon : Sum  Inputs=+-
  error_1L_Ad : Sum
  error_1L_Convert : DataTypeConversion  OutDataTypeStr=uint32
  error_1L_F : Gain
  error_1L_L : simulink/Logic and Bit Operations/Bitwise Operator  logicop=AND  UseBitMask=on  BitMask=65535  BitMaskRealWorld=Stored Integer
  error_1L_O : Constant  Value=0  OutDataTypeStr=single
  error_1L_S : ArithShift
  error_1L_Sub : Subsystem
  error_1L_sat : Saturate  UpperLimit=65535  LowerLimit=0
  error_1Lcv : DataTypeConversion
  error_1Linput6_Ad : Sum
  error_1Linput6_C : Constant  Value=256
  error_1Linput6_P : Product
  IGBT_1L_Out : Outport
  error_1L_Out : Outport  Port=2
  Inv_1L_Out : Outport  Port=3
  Mot_1L_Out : Outport  Port=4
  wires:
  input/1 -> Demux/1
  Mot_1LROP/1 -> Mot_1LSW/2
  Mot_1LSW/1 -> Mot_1L_F/1
  Mot_1LMinus/1 -> Mot_1LSW/1
  Mot_1Lsubcon/1 -> Mot_1LMinus/1
  Mot_1LCS/1 -> Mot_1Lsubcon/1
  Mot_1LCS1/1 -> Mot_1LROP/2
  Mot_1LConS/1 -> Mot_1LCS1/1, Mot_1LCS/1
  Mot_1Lcv/1 -> Mot_1LSW/3, Mot_1Lsubcon/2, Mot_1LROP/1
  Mot_1L_S/1 -> Mot_1Lcv/1
  Mot_1L_L/1 -> Mot_1L_S/1
  Mot_1L_Convert/1 -> Mot_1L_L/1
  Mot_1L_Sub/1(Out1) -> Mot_1L_Convert/1
  Mot_1Linput2_Ad/1 -> Mot_1L_Sub/1(In1)
  Demux/1 -> Mot_1Linput2_Ad/2
  Mot_1Linput2_P/1 -> Mot_1Linput2_Ad/1
  Mot_1Linput2_C/1 -> Mot_1Linput2_P/2
  Demux/2 -> Mot_1Linput2_P/1
  Mot_1L_sat/1 -> Mot_1L_Out/1
  Mot_1L_Ad/1 -> Mot_1L_sat/1
  Mot_1L_O/1 -> Mot_1L_Ad/2
  Mot_1L_F/1 -> Mot_1L_Ad/1
  Inv_1LROP/1 -> Inv_1LSW/2
  Inv_1LSW/1 -> Inv_1L_F/1
  Inv_1LMinus/1 -> Inv_1LSW/1
  Inv_1Lsubcon/1 -> Inv_1LMinus/1
  Inv_1LCS/1 -> Inv_1Lsubcon/1
  Inv_1LCS1/1 -> Inv_1LROP/2
  Inv_1LConS/1 -> Inv_1LCS1/1, Inv_1LCS/1
  Inv_1Lcv/1 -> Inv_1Lsubcon/2, Inv_1LROP/1, Inv_1LSW/3
  Inv_1L_S/1 -> Inv_1Lcv/1
  Inv_1L_L/1 -> Inv_1L_S/1
  Inv_1L_Convert/1 -> Inv_1L_L/1
  Inv_1L_Sub/1(Out1) -> Inv_1L_Convert/1
  Inv_1Linput4_Ad/1 -> Inv_1L_Sub/1(In1)
  Demux/3 -> Inv_1Linput4_Ad/2
  Inv_1Linput4_P/1 -> Inv_1Linput4_Ad/1
  Inv_1Linput4_C/1 -> Inv_1Linput4_P/2
  Demux/4 -> Inv_1Linput4_P/1
  Inv_1L_sat/1 -> Inv_1L_Out/1
  Inv_1L_Ad/1 -> Inv_1L_sat/1
  Inv_1L_O/1 -> Inv_1L_Ad/2
  Inv_1L_F/1 -> Inv_1L_Ad/1
  error_1Lcv/1 -> error_1L_F/1
  error_1L_S/1 -> error_1Lcv/1
  error_1L_L/1 -> error_1L_S/1
  error_1L_Convert/1 -> error_1L_L/1
  error_1L_Sub/1(Out1) -> error_1L_Convert/1
  error_1Linput6_Ad/1 -> error_1L_Sub/1(In1)
  Demux/5 -> error_1Linput6_Ad/2
  error_1Linput6_P/1 -> error_1Linput6_Ad/1
  error_1Linput6_C/1 -> error_1Linput6_P/2
  Demux/6 -> error_1Linput6_P/1
  error_1L_sat/1 -> error_1L_Out/1
  error_1L_Ad/1 -> error_1L_sat/1
  error_1L_O/1 -> error_1L_Ad/2
  error_1L_F/1 -> error_1L_Ad/1
  IGBT_1LROP/1 -> IGBT_1LSW/2
  IGBT_1LSW/1 -> IGBT_1L_F/1
  IGBT_1LMinus/1 -> IGBT_1LSW/1
  IGBT_1Lsubcon/1 -> IGBT_1LMinus/1
  IGBT_1LCS/1 -> IGBT_1Lsubcon/1
  IGBT_1LCS1/1 -> IGBT_1LROP/2
  IGBT_1LConS/1 -> IGBT_1LCS1/1, IGBT_1LCS/1
  IGBT_1Lcv/1 -> IGBT_1Lsubcon/2, IGBT_1LROP/1, IGBT_1LSW/3
  IGBT_1L_S/1 -> IGBT_1Lcv/1
  IGBT_1L_L/1 -> IGBT_1L_S/1
  IGBT_1L_Convert/1 -> IGBT_1L_L/1
  IGBT_1L_Sub/1(Out1) -> IGBT_1L_Convert/1
  IGBT_1Linput8_Ad/1 -> IGBT_1L_Sub/1(In1)
  Demux/7 -> IGBT_1Linput8_Ad/2
  IGBT_1Linput8_P/1 -> IGBT_1Linput8_Ad/1
  IGBT_1Linput8_C/1 -> IGBT_1Linput8_P/2
  Demux/8 -> IGBT_1Linput8_P/1
  IGBT_1L_sat/1 -> IGBT_1L_Out/1
  IGBT_1L_Ad/1 -> IGBT_1L_sat/1
  IGBT_1L_O/1 -> IGBT_1L_Ad/2
  IGBT_1L_F/1 -> IGBT_1L_Ad/1

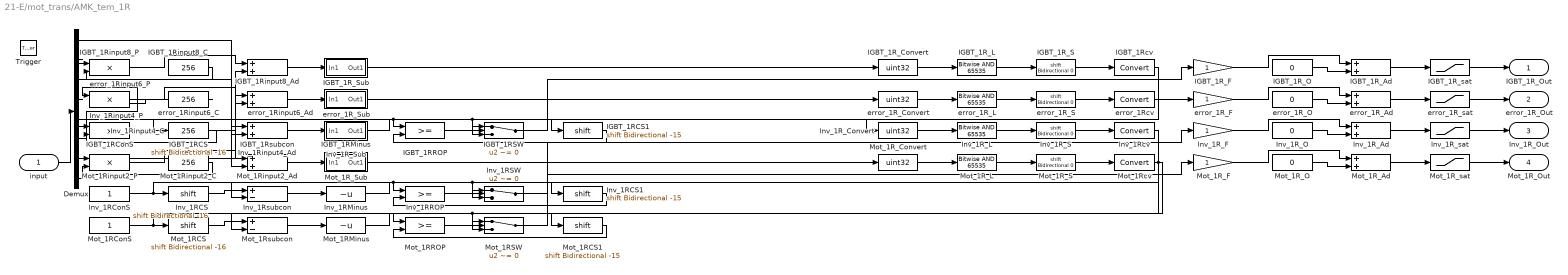
== system 21-E/mot_trans/AMK_tem_1R ==
  input : Inport
  Trigger : TriggerPort  TriggerType=function-call  PortDimensions=1
  Demux : Demux  Outputs=8
  IGBT_1RCS : ArithShift  BitShiftNumber=-16
  IGBT_1RCS1 : ArithShift  BitShiftNumber=-15
  IGBT_1RConS : Constant  OutDataTypeStr=single
  IGBT_1RMinus : UnaryMinus
  IGBT_1RROP : RelationalOperator  OutDataTypeStr=boolean
  IGBT_1RSW : Switch  Criteria=u2 ~= 0
  IGBT_1R_Ad : Sum
  IGBT_1R_Convert : DataTypeConversion  OutDataTypeStr=uint32
  IGBT_1R_F : Gain
  IGBT_1R_L : simulink/Logic and Bit Operations/Bitwise Operator  logicop=AND  UseBitMask=on  BitMask=65535  BitMaskRealWorld=Stored Integer
  IGBT_1R_O : Constant  Value=0  OutDataTypeStr=single
  IGBT_1R_S : ArithShift
  IGBT_1R_Sub : Subsystem
  IGBT_1R_sat : Saturate  UpperLimit=32767  LowerLimit=-32768
  IGBT_1Rcv : DataTypeConversion
  IGBT_1Rinput8_Ad : Sum
  IGBT_1Rinput8_C : Constant  Value=256
  IGBT_1Rinput8_P : Product
  IGBT_1Rsubcon : Sum  Inputs=+-
  Inv_1RCS : ArithShift  BitShiftNumber=-16
  Inv_1RCS1 : ArithShift  BitShiftNumber=-15
  Inv_1RConS : Constant  OutDataTypeStr=single
  Inv_1RMinus : UnaryMinus
  Inv_1RROP : RelationalOperator  OutDataTypeStr=boolean
  Inv_1RSW : Switch  Criteria=u2 ~= 0
  Inv_1R_Ad : Sum
  Inv_1R_Convert : DataTypeConversion  OutDataTypeStr=uint32
  Inv_1R_F : Gain
  Inv_1R_L : simulink/Logic and Bit Operations/Bitwise Operator  logicop=AND  UseBitMask=on  BitMask=65535  BitMaskRealWorld=Stored Integer
  Inv_1R_O : Constant  Value=0  OutDataTypeStr=single
  Inv_1R_S : ArithShift
  Inv_1R_Sub : Subsystem
  Inv_1R_sat : Saturate  UpperLimit=32767  LowerLimit=-32768
  Inv_1Rcv : DataTypeConversion
  Inv_1Rinput4_Ad : Sum
  Inv_1Rinput4_C : Constant  Value=256
  Inv_1Rinput4_P : Product
  Inv_1Rsubcon : Sum  Inputs=+-
  Mot_1RCS : ArithShift  BitShiftNumber=-16
  Mot_1RCS1 : ArithShift  BitShiftNumber=-15
  Mot_1RConS : Constant  OutDataTypeStr=single
  Mot_1RMinus : UnaryMinus
  Mot_1RROP : RelationalOperator  OutDataTypeStr=boolean
  Mot_1RSW : Switch  Criteria=u2 ~= 0
  Mot_1R_Ad : Sum
  Mot_1R_Convert : DataTypeConversion  OutDataTypeStr=uint32
  Mot_1R_F : Gain
  Mot_1R_L : simulink/Logic and Bit Operations/Bitwise Operator  logicop=AND  UseBitMask=on  BitMask=65535  BitMaskRealWorld=Stored Integer
  Mot_1R_O : Constant  Value=0  OutDataTypeStr=single
  Mot_1R_S : ArithShift
  Mot_1R_Sub : Subsystem
  Mot_1R_sat : Saturate  UpperLimit=32767  LowerLimit=-32768
  Mot_1Rcv : DataTypeConversion
  Mot_1Rinput2_Ad : Sum
  Mot_1Rinput2_C : Constant  Value=256
  Mot_1Rinput2_P : Product
  Mot_1Rsubcon : Sum  Inputs=+-
  error_1R_Ad : Sum
  error_1R_Convert : DataTypeConversion  OutDataTypeStr=uint32
  error_1R_F : Gain
  error_1R_L : simulink/Logic and Bit Operations/Bitwise Operator  logicop=AND  UseBitMask=on  BitMask=65535  BitMaskRealWorld=Stored Integer
  error_1R_O : Constant  Value=0  OutDataTypeStr=single
  error_1R_S : ArithShift
  error_1R_Sub : Subsystem
  error_1R_sat : Saturate  UpperLimit=65535  LowerLimit=0
  error_1Rcv : DataTypeConversion
  error_1Rinput6_Ad : Sum
  error_1Rinput6_C : Constant  Value=256
  error_1Rinput6_P : Product
  IGBT_1R_Out : Outport
  error_1R_Out : Outport  Port=2
  Inv_1R_Out : Outport  Port=3
  Mot_1R_Out : Outport  Port=4
  wires:
  input/1 -> Demux/1
  Mot_1RROP/1 -> Mot_1RSW/2
  Mot_1RSW/1 -> Mot_1R_F/1
  Mot_1RMinus/1 -> Mot_1RSW/1
  Mot_1Rsubcon/1 -> Mot_1RMinus/1
  Mot_1RCS/1 -> Mot_1Rsubcon/1
  Mot_1RCS1/1 -> Mot_1RROP/2
  Mot_1RConS/1 -> Mot_1RCS1/1, Mot_1RCS/1
  Mot_1Rcv/1 -> Mot_1RSW/3, Mot_1Rsubcon/2, Mot_1RROP/1
  Mot_1R_S/1 -> Mot_1Rcv/1
  Mot_1R_L/1 -> Mot_1R_S/1
  Mot_1R_Convert/1 -> Mot_1R_L/1
  Mot_1R_Sub/1(Out1) -> Mot_1R_Convert/1
  Mot_1Rinput2_Ad/1 -> Mot_1R_Sub/1(In1)
  Demux/1 -> Mot_1Rinput2_Ad/2
  Mot_1Rinput2_P/1 -> Mot_1Rinput2_Ad/1
  Mot_1Rinput2_C/1 -> Mot_1Rinput2_P/2
  Demux/2 -> Mot_1Rinput2_P/1
  Mot_1R_sat/1 -> Mot_1R_Out/1
  Mot_1R_Ad/1 -> Mot_1R_sat/1
  Mot_1R_O/1 -> Mot_1R_Ad/2
  Mot_1R_F/1 -> Mot_1R_Ad/1
  Inv_1RROP/1 -> Inv_1RSW/2
  Inv_1RSW/1 -> Inv_1R_F/1
  Inv_1RMinus/1 -> Inv_1RSW/1
  Inv_1Rsubcon/1 -> Inv_1RMinus/1
  Inv_1RCS/1 -> Inv_1Rsubcon/1
  Inv_1RCS1/1 -> Inv_1RROP/2
  Inv_1RConS/1 -> Inv_1RCS1/1, Inv_1RCS/1
  Inv_1Rcv/1 -> Inv_1Rsubcon/2, Inv_1RROP/1, Inv_1RSW/3
  Inv_1R_S/1 -> Inv_1Rcv/1
  Inv_1R_L/1 -> Inv_1R_S/1
  Inv_1R_Convert/1 -> Inv_1R_L/1
  Inv_1R_Sub/1(Out1) -> Inv_1R_Convert/1
  Inv_1Rinput4_Ad/1 -> Inv_1R_Sub/1(In1)
  Demux/3 -> Inv_1Rinput4_Ad/2
  Inv_1Rinput4_P/1 -> Inv_1Rinput4_Ad/1
  Inv_1Rinput4_C/1 -> Inv_1Rinput4_P/2
  Demux/4 -> Inv_1Rinput4_P/1
  Inv_1R_sat/1 -> Inv_1R_Out/1
  Inv_1R_Ad/1 -> Inv_1R_sat/1
  Inv_1R_O/1 -> Inv_1R_Ad/2
  Inv_1R_F/1 -> Inv_1R_Ad/1
  error_1Rcv/1 -> error_1R_F/1
  error_1R_S/1 -> error_1Rcv/1
  error_1R_L/1 -> error_1R_S/1
  error_1R_Convert/1 -> error_1R_L/1
  error_1R_Sub/1(Out1) -> error_1R_Convert/1
  error_1Rinput6_Ad/1 -> error_1R_Sub/1(In1)
  Demux/5 -> error_1Rinput6_Ad/2
  error_1Rinput6_P/1 -> error_1Rinput6_Ad/1
  error_1Rinput6_C/1 -> error_1Rinput6_P/2
  Demux/6 -> error_1Rinput6_P/1
  error_1R_sat/1 -> error_1R_Out/1
  error_1R_Ad/1 -> error_1R_sat/1
  error_1R_O/1 -> error_1R_Ad/2
  error_1R_F/1 -> error_1R_Ad/1
  IGBT_1RROP/1 -> IGBT_1RSW/2
  IGBT_1RSW/1 -> IGBT_1R_F/1
  IGBT_1RMinus/1 -> IGBT_1RSW/1
  IGBT_1Rsubcon/1 -> IGBT_1RMinus/1
  IGBT_1RCS/1 -> IGBT_1Rsubcon/1
  IGBT_1RCS1/1 -> IGBT_1RROP/2
  IGBT_1RConS/1 -> IGBT_1RCS1/1, IGBT_1RCS/1
  IGBT_1Rcv/1 -> IGBT_1Rsubcon/2, IGBT_1RROP/1, IGBT_1RSW/3
  IGBT_1R_S/1 -> IGBT_1Rcv/1
  IGBT_1R_L/1 -> IGBT_1R_S/1
  IGBT_1R_Convert/1 -> IGBT_1R_L/1
  IGBT_1R_Sub/1(Out1) -> IGBT_1R_Convert/1
  IGBT_1Rinput8_Ad/1 -> IGBT_1R_Sub/1(In1)
  Demux/7 -> IGBT_1Rinput8_Ad/2
  IGBT_1Rinput8_P/1 -> IGBT_1Rinput8_Ad/1
  IGBT_1Rinput8_C/1 -> IGBT_1Rinput8_P/2
  Demux/8 -> IGBT_1Rinput8_P/1
  IGBT_1R_sat/1 -> IGBT_1R_Out/1
  IGBT_1R_Ad/1 -> IGBT_1R_sat/1
  IGBT_1R_O/1 -> IGBT_1R_Ad/2
  IGBT_1R_F/1 -> IGBT_1R_Ad/1

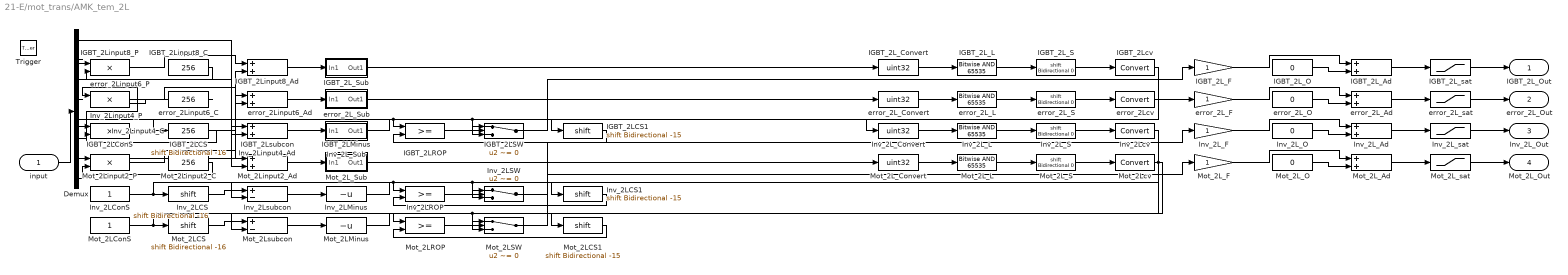
== system 21-E/mot_trans/AMK_tem_2L ==
  input : Inport
  Trigger : TriggerPort  TriggerType=function-call  PortDimensions=1
  Demux : Demux  Outputs=8
  IGBT_2LCS : ArithShift  BitShiftNumber=-16
  IGBT_2LCS1 : ArithShift  BitShiftNumber=-15
  IGBT_2LConS : Constant  OutDataTypeStr=single
  IGBT_2LMinus : UnaryMinus
  IGBT_2LROP : RelationalOperator  OutDataTypeStr=boolean
  IGBT_2LSW : Switch  Criteria=u2 ~= 0
  IGBT_2L_Ad : Sum
  IGBT_2L_Convert : DataTypeConversion  OutDataTypeStr=uint32
  IGBT_2L_F : Gain
  IGBT_2L_L : simulink/Logic and Bit Operations/Bitwise Operator  logicop=AND  UseBitMask=on  BitMask=65535  BitMaskRealWorld=Stored Integer
  IGBT_2L_O : Constant  Value=0  OutDataTypeStr=single
  IGBT_2L_S : ArithShift
  IGBT_2L_Sub : Subsystem
  IGBT_2L_sat : Saturate  UpperLimit=32767  LowerLimit=-32768
  IGBT_2Lcv : DataTypeConversion
  IGBT_2Linput8_Ad : Sum
  IGBT_2Linput8_C : Constant  Value=256
  IGBT_2Linput8_P : Product
  IGBT_2Lsubcon : Sum  Inputs=+-
  Inv_2LCS : ArithShift  BitShiftNumber=-16
  Inv_2LCS1 : ArithShift  BitShiftNumber=-15
  Inv_2LConS : Constant  OutDataTypeStr=single
  Inv_2LMinus : UnaryMinus
  Inv_2LROP : RelationalOperator  OutDataTypeStr=boolean
  Inv_2LSW : Switch  Criteria=u2 ~= 0
  Inv_2L_Ad : Sum
  Inv_2L_Convert : DataTypeConversion  OutDataTypeStr=uint32
  Inv_2L_F : Gain
  Inv_2L_L : simulink/Logic and Bit Operations/Bitwise Operator  logicop=AND  UseBitMask=on  BitMask=65535  BitMaskRealWorld=Stored Integer
  Inv_2L_O : Constant  Value=0  OutDataTypeStr=single
  Inv_2L_S : ArithShift
  Inv_2L_Sub : Subsystem
  Inv_2L_sat : Saturate  UpperLimit=32767  LowerLimit=-32768
  Inv_2Lcv : DataTypeConversion
  Inv_2Linput4_Ad : Sum
  Inv_2Linput4_C : Constant  Value=256
  Inv_2Linput4_P : Product
  Inv_2Lsubcon : Sum  Inputs=+-
  Mot_2LCS : ArithShift  BitShiftNumber=-16
  Mot_2LCS1 : ArithShift  BitShiftNumber=-15
  Mot_2LConS : Constant  OutDataTypeStr=single
  Mot_2LMinus : UnaryMinus
  Mot_2LROP : RelationalOperator  OutDataTypeStr=boolean
  Mot_2LSW : Switch  Criteria=u2 ~= 0
  Mot_2L_Ad : Sum
  Mot_2L_Convert : DataTypeConversion  OutDataTypeStr=uint32
  Mot_2L_F : Gain
  Mot_2L_L : simulink/Logic and Bit Operations/Bitwise Operator  logicop=AND  UseBitMask=on  BitMask=65535  BitMaskRealWorld=Stored Integer
  Mot_2L_O : Constant  Value=0  OutDataTypeStr=single
  Mot_2L_S : ArithShift
  Mot_2L_Sub : Subsystem
  Mot_2L_sat : Saturate  UpperLimit=32767  LowerLimit=-32768
  Mot_2Lcv : DataTypeConversion
  Mot_2Linput2_Ad : Sum
  Mot_2Linput2_C : Constant  Value=256
  Mot_2Linput2_P : Product
  Mot_2Lsubcon : Sum  Inputs=+-
  error_2L_Ad : Sum
  error_2L_Convert : DataTypeConversion  OutDataTypeStr=uint32
  error_2L_F : Gain
  error_2L_L : simulink/Logic and Bit Operations/Bitwise Operator  logicop=AND  UseBitMask=on  BitMask=65535  BitMaskRealWorld=Stored Integer
  error_2L_O : Constant  Value=0  OutDataTypeStr=single
  error_2L_S : ArithShift
  error_2L_Sub : Subsystem
  error_2L_sat : Saturate  UpperLimit=65535  LowerLimit=0
  error_2Lcv : DataTypeConversion
  error_2Linput6_Ad : Sum
  error_2Linput6_C : Constant  Value=256
  error_2Linput6_P : Product
  IGBT_2L_Out : Outport
  error_2L_Out : Outport  Port=2
  Inv_2L_Out : Outport  Port=3
  Mot_2L_Out : Outport  Port=4
  wires:
  input/1 -> Demux/1
  Mot_2LROP/1 -> Mot_2LSW/2
  Mot_2LSW/1 -> Mot_2L_F/1
  Mot_2LMinus/1 -> Mot_2LSW/1
  Mot_2Lsubcon/1 -> Mot_2LMinus/1
  Mot_2LCS/1 -> Mot_2Lsubcon/1
  Mot_2LCS1/1 -> Mot_2LROP/2
  Mot_2LConS/1 -> Mot_2LCS1/1, Mot_2LCS/1
  Mot_2Lcv/1 -> Mot_2LSW/3, Mot_2Lsubcon/2, Mot_2LROP/1
  Mot_2L_S/1 -> Mot_2Lcv/1
  Mot_2L_L/1 -> Mot_2L_S/1
  Mot_2L_Convert/1 -> Mot_2L_L/1
  Mot_2L_Sub/1(Out1) -> Mot_2L_Convert/1
  Mot_2Linput2_Ad/1 -> Mot_2L_Sub/1(In1)
  Demux/1 -> Mot_2Linput2_Ad/2
  Mot_2Linput2_P/1 -> Mot_2Linput2_Ad/1
  Mot_2Linput2_C/1 -> Mot_2Linput2_P/2
  Demux/2 -> Mot_2Linput2_P/1
  Mot_2L_sat/1 -> Mot_2L_Out/1
  Mot_2L_Ad/1 -> Mot_2L_sat/1
  Mot_2L_O/1 -> Mot_2L_Ad/2
  Mot_2L_F/1 -> Mot_2L_Ad/1
  Inv_2LROP/1 -> Inv_2LSW/2
  Inv_2LSW/1 -> Inv_2L_F/1
  Inv_2LMinus/1 -> Inv_2LSW/1
  Inv_2Lsubcon/1 -> Inv_2LMinus/1
  Inv_2LCS/1 -> Inv_2Lsubcon/1
  Inv_2LCS1/1 -> Inv_2LROP/2
  Inv_2LConS/1 -> Inv_2LCS1/1, Inv_2LCS/1
  Inv_2Lcv/1 -> Inv_2Lsubcon/2, Inv_2LROP/1, Inv_2LSW/3
  Inv_2L_S/1 -> Inv_2Lcv/1
  Inv_2L_L/1 -> Inv_2L_S/1
  Inv_2L_Convert/1 -> Inv_2L_L/1
  Inv_2L_Sub/1(Out1) -> Inv_2L_Convert/1
  Inv_2Linput4_Ad/1 -> Inv_2L_Sub/1(In1)
  Demux/3 -> Inv_2Linput4_Ad/2
  Inv_2Linput4_P/1 -> Inv_2Linput4_Ad/1
  Inv_2Linput4_C/1 -> Inv_2Linput4_P/2
  Demux/4 -> Inv_2Linput4_P/1
  Inv_2L_sat/1 -> Inv_2L_Out/1
  Inv_2L_Ad/1 -> Inv_2L_sat/1
  Inv_2L_O/1 -> Inv_2L_Ad/2
  Inv_2L_F/1 -> Inv_2L_Ad/1
  error_2Lcv/1 -> error_2L_F/1
  error_2L_S/1 -> error_2Lcv/1
  error_2L_L/1 -> error_2L_S/1
  error_2L_Convert/1 -> error_2L_L/1
  error_2L_Sub/1(Out1) -> error_2L_Convert/1
  error_2Linput6_Ad/1 -> error_2L_Sub/1(In1)
  Demux/5 -> error_2Linput6_Ad/2
  error_2Linput6_P/1 -> error_2Linput6_Ad/1
  error_2Linput6_C/1 -> error_2Linput6_P/2
  Demux/6 -> error_2Linput6_P/1
  error_2L_sat/1 -> error_2L_Out/1
  error_2L_Ad/1 -> error_2L_sat/1
  error_2L_O/1 -> error_2L_Ad/2
  error_2L_F/1 -> error_2L_Ad/1
  IGBT_2LROP/1 -> IGBT_2LSW/2
  IGBT_2LSW/1 -> IGBT_2L_F/1
  IGBT_2LMinus/1 -> IGBT_2LSW/1
  IGBT_2Lsubcon/1 -> IGBT_2LMinus/1
  IGBT_2LCS/1 -> IGBT_2Lsubcon/1
  IGBT_2LCS1/1 -> IGBT_2LROP/2
  IGBT_2LConS/1 -> IGBT_2LCS1/1, IGBT_2LCS/1
  IGBT_2Lcv/1 -> IGBT_2Lsubcon/2, IGBT_2LROP/1, IGBT_2LSW/3
  IGBT_2L_S/1 -> IGBT_2Lcv/1
  IGBT_2L_L/1 -> IGBT_2L_S/1
  IGBT_2L_Convert/1 -> IGBT_2L_L/1
  IGBT_2L_Sub/1(Out1) -> IGBT_2L_Convert/1
  IGBT_2Linput8_Ad/1 -> IGBT_2L_Sub/1(In1)
  Demux/7 -> IGBT_2Linput8_Ad/2
  IGBT_2Linput8_P/1 -> IGBT_2Linput8_Ad/1
  IGBT_2Linput8_C/1 -> IGBT_2Linput8_P/2
  Demux/8 -> IGBT_2Linput8_P/1
  IGBT_2L_sat/1 -> IGBT_2L_Out/1
  IGBT_2L_Ad/1 -> IGBT_2L_sat/1
  IGBT_2L_O/1 -> IGBT_2L_Ad/2
  IGBT_2L_F/1 -> IGBT_2L_Ad/1
